simulink model "Motor_Pos"  (R2023b)
settings: Solver=ode15s  StartTime=0.0  StopTime=20  RelTol=1e-3
values from neighbouring files (symbols this model uses):
  b = 1.264E-4    (= 0.0001264)    [motor_parameters.m]
  J = 7.89E-2    (= 0.0789)    [motor_parameters.m]
  Km = 0.8878    [motor_parameters.m]
  L = 3.2E-3    (= 0.0032)    [motor_parameters.m]
  R = 6.2    [motor_parameters.m]
settings Model: Creator=sansh  LastModifiedBy=Jayden
settings SolverCC: AlgebraicLoopSolver=TrustRegion
settings DataIOCC: ReturnWorkspaceOutputs=off
settings DebuggingCC: UnconnectedInputMsg=warning  UnconnectedOutputMsg=warning  UnconnectedLineMsg=warning  ArithmeticOperatorsInVariantConditions=warning
settings ModelReferenceCC: EnableRefExpFcnMdlSchedulingChecks=on
settings SFSimCC: SimUseLocalCustomCode=off  CustomCodeUndefinedFunction=UseInterfaceOnly
settings RTWCC: RTWUseLocalCustomCode=off
settings CodeAppCC: StateflowObjectComments=on

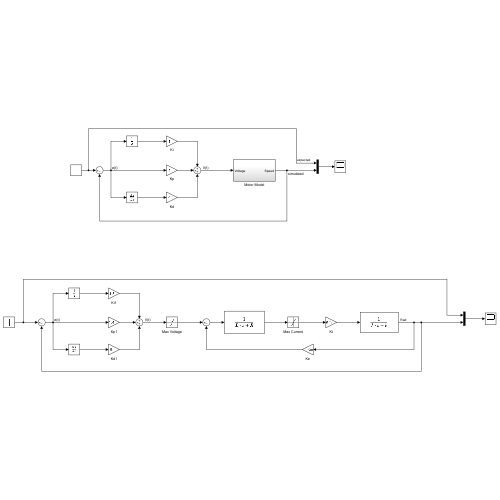
[thumbnail: Simulink's stored preview of the top-level diagram]
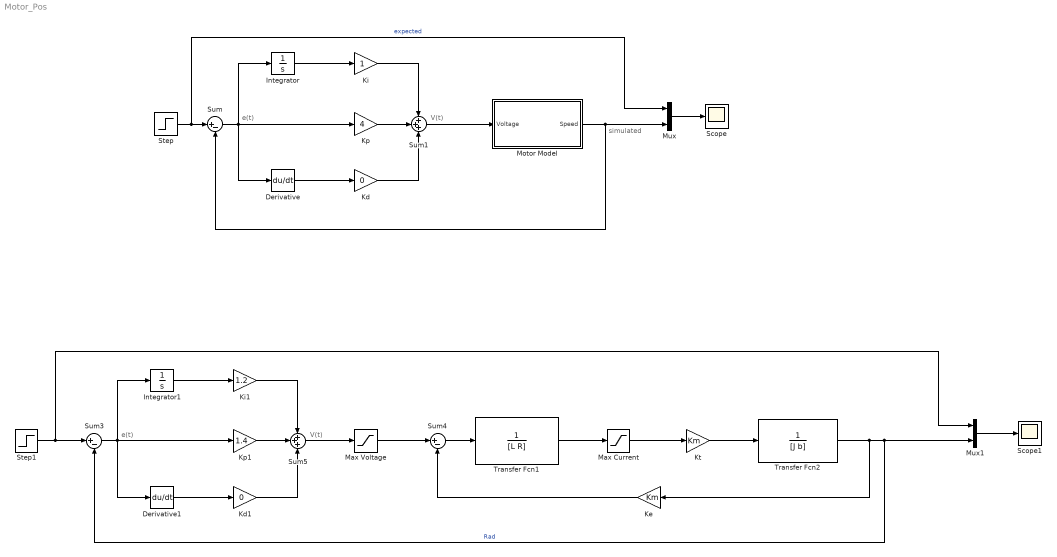
== system Motor_Pos ==
  note: simulated
  note: V(t)
  note: e(t)
  note: e(t)
  note: V(t)
  Derivative : Derivative
  Derivative1 : Derivative
  Integrator : Integrator
  Integrator1 : Integrator
  Kd : Gain  Gain=0
  Kd1 : Gain  Gain=0
  Ke : Gain  Gain=Km
  Ki : Gain
  Ki1 : Gain  Gain=1.2
  Kp : Gain  Gain=4
  Kp1 : Gain  Gain=1.4
  Kt : Gain  Gain=Km
  Max Current : Saturate  UpperLimit=0.3  LowerLimit=0
  Max Voltage : Saturate  UpperLimit=12  LowerLimit=0
  Motor Model : Subsystem
  Mux : Mux  Inputs=2
  Mux1 : Mux  Inputs=2
  Scope : Scope
  Scope1 : Scope
  Step : Step  SampleTime=0
  Step1 : Step  SampleTime=0
  Sum : Sum  Inputs=|+-
  Sum1 : Sum  Inputs=+++
  Sum3 : Sum  Inputs=|+-
  Sum4 : Sum  Inputs=|+-
  Sum5 : Sum  Inputs=+++
  Transfer Fcn1 : TransferFcn  Denominator=[L R]
  Transfer Fcn2 : TransferFcn  Denominator=[J b]
  wires:
  Sum1/1 -> Motor Model/1(Voltage)
  Step/1 -> Mux/1, Sum/1  "expected"
  Sum/1 -> Derivative/1, Integrator/1, Kp/1
  Kp/1 -> Sum1/2
  Ki/1 -> Sum1/1
  Kd/1 -> Sum1/3
  Mux/1 -> Scope/1
  Integrator/1 -> Ki/1
  Derivative/1 -> Kd/1
  Motor Model/1(Speed) -> Mux/2, Sum/2
  Kt/1 -> Transfer Fcn2/1
  Sum4/1 -> Transfer Fcn1/1
  Ke/1 -> Sum4/2
  Transfer Fcn1/1 -> Max Current/1
  Max Current/1 -> Kt/1
  Mux1/1 -> Scope1/1
  Derivative1/1 -> Kd1/1
  Step1/1 -> Mux1/1, Sum3/1
  Sum5/1 -> Max Voltage/1
  Kp1/1 -> Sum5/2
  Kd1/1 -> Sum5/3
  Ki1/1 -> Sum5/1
  Integrator1/1 -> Ki1/1
  Sum3/1 -> Derivative1/1, Integrator1/1, Kp1/1
  Transfer Fcn2/1 -> Mux1/2, Sum3/2, Ke/1  "Rad"
  Max Voltage/1 -> Sum4/1

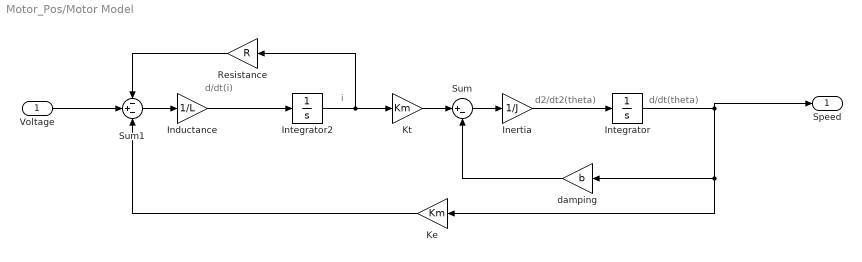
== system Motor_Pos/Motor Model ==
  note: i
  note: d/dt(i)
  note: d2/dt2(theta)
  note: d/dt(theta)
  Voltage : Inport
  Inductance : Gain  Gain=1/L
  Inertia : Gain  Gain=1/J
  Integrator : Integrator
  Integrator2 : Integrator
  Ke : Gain  Gain=Km
  Kt : Gain  Gain=Km
  Resistance : Gain  Gain=R
  Sum : Sum  Inputs=|+-
  Sum1 : Sum  Inputs=-+-
  damping : Gain  Gain=b
  Speed : Outport
  wires:
  Inertia/1 -> Integrator/1
  Inductance/1 -> Integrator2/1
  Integrator2/1 -> Resistance/1, Kt/1
  Integrator/1 -> damping/1, Ke/1, Speed/1
  damping/1 -> Sum/2
  Kt/1 -> Sum/1
  Sum/1 -> Inertia/1
  Resistance/1 -> Sum1/1
  Sum1/1 -> Inductance/1
  Ke/1 -> Sum1/3
  Voltage/1 -> Sum1/2
